simulink model "modFer"  (R2016b)
settings: Solver=VariableStepAuto  StartTime=0.0  StopTime=20  RelTol=1e-3  EnableMultiTasking=on
values from neighbouring files (symbols this model uses):
  A = [ 0   0  0 ... (first row only)    [detectability.m]    (also in param.m = [-0.02   1    1)
  B = [1.6;0.23;0]    [param.m]
  C = [ 0 0 0]    [detectability.m]    (also in param.m = [1 0 0])
  Ci = eye(3)    [param.m]
  D = zeros(1,1)    [param.m]
  K1lqr = Klqr(1:3)    [param.m]
  Kslqr = Klqr(4)    [param.m]
settings Model: Creator=ganou2u  LastModifiedBy=arek
settings OptimizationCC: LifeSpan=inf
settings DebuggingCC: SFUnexpectedBacktrackingDiag=warning  SFNoUnconditionalDefaultTransitionDiag=warning  SFExecutionAtInitializationDiag=none
settings GRTTargetCC: TargetLangStandard=C89/C90 (ANSI)  GeneratePreprocessorConditionals=Disable all
settings ConfigComp: CovMetricSettings=dw  CovHtmlReporting=on  CovSaveCumulativeToWorkspaceVar=on  CovSaveSingleToWorkspaceVar=on  CovExternalEMLEnable=off

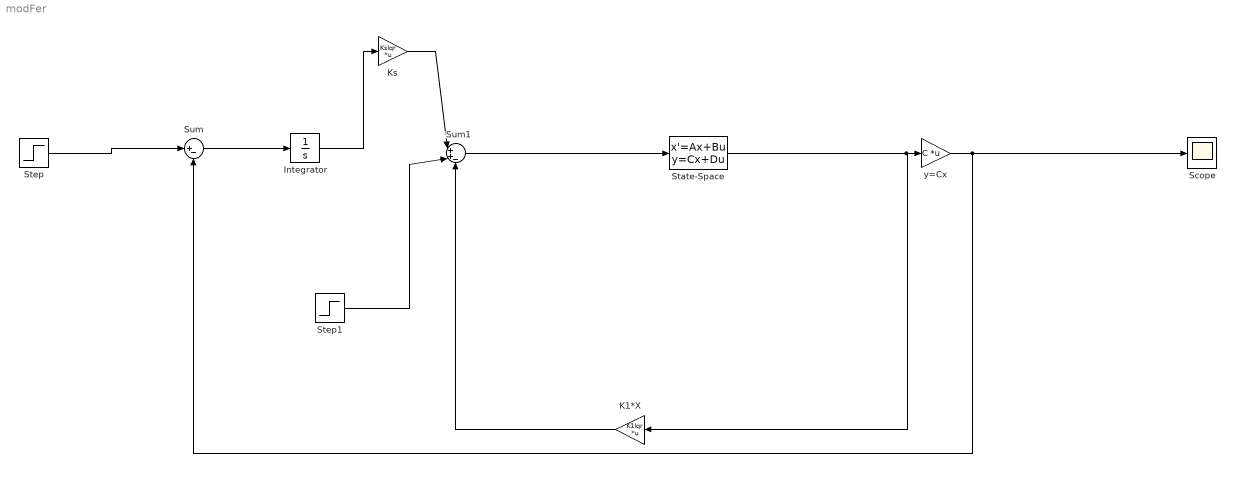
== system modFer ==
  "\ty=Cx" : Gain  Gain=C  Multiplication=Matrix(K*u)
  Integrator : Integrator
  K1*X : Gain  Gain=K1lqr  Multiplication=Matrix(K*u)
  Ks : Gain  Gain=Kslqr  Multiplication=Matrix(K*u)
  Scope : Scope
  State-Space : StateSpace  A=A  B=B  C=Ci  D=D  X0=0
  Step : Step  Time=0  SampleTime=0
  Step1 : Step  Time=80  After=20  SampleTime=0
  Sum : Sum  Inputs=|+-
  Sum1 : Sum  Inputs=|++-
  wires:
  Step/1 -> Sum/1
  "\ty=Cx"/1 -> Sum/2, Scope/1
  State-Space/1 -> K1*X/1, "\ty=Cx"/1
  Sum1/1 -> State-Space/1
  Sum/1 -> Integrator/1
  Integrator/1 -> Ks/1
  Ks/1 -> Sum1/1
  K1*X/1 -> Sum1/3
  Step1/1 -> Sum1/2
